simulink model "X8_trim"  (R2020a)
settings: Solver=ode45  StartTime=0.0  StopTime=20.0  RelTol=1e-4  EnableMultiTasking=on
values from neighbouring files (symbols this model uses):
  C_L_delta_eInterpolation = Create_interpolation(C_L_delta_e_data,'C_L_delta_e_data')    [coeff_ctrl.m]
  P = filter.P(i,i,k_0:k_1)    [filterTest.m]    (also in kalmanFilters.m = oldFilter.P(:,:,k))
  T_elevon2ailelev = [1 1 ... (first row only)    [init.m]
  x0 = X_trim    [X8Trim.m]    (also in init.m = [eta_0', ny_0' zeros(1,6)]'; runX8.m = [      0                 0                    -h_ini        ; trimX8.m = [      37.5                 0                    -h_ini     )
libraries: aerolibactuator x3
settings Model: Creator=krisgry  LastModifiedBy=olema
settings DataIOCC: LimitDataPoints=on  SaveFormat=Array  ReturnWorkspaceOutputs=off
settings OptimizationCC: LifeSpan=inf
settings DebuggingCC: SolverPrmCheckMsg=warning  SFUnexpectedBacktrackingDiag=warning  SFNoUnconditionalDefaultTransitionDiag=warning  SFExecutionAtInitializationDiag=none  UnderSpecifiedDimensionMsg=warning  ArithmeticOperatorsInVariantConditions=warning
settings HardwareCC: ProdBitPerPointer=32  ProdBitPerSizeT=32  ProdBitPerPtrDiffT=32  ProdLargestAtomicFloat=None  ProdIntDivRoundTo=Undefined  ProdEndianess=Unspecified  ProdWordSize=32  ProdHWDeviceType=32-bit Generic
settings ModelReferenceCC: PropagateSignalLabelsOutOfModel=off
settings SFSimCC: SimUseLocalCustomCode=off  CustomCodeUndefinedFunction=UseInterfaceOnly
settings RTWCC: RTWUseLocalCustomCode=off
settings CodeAppCC: StateflowObjectComments=on
settings GRTTargetCC: TargetLangStandard=C89/C90 (ANSI)
settings ConfigComp: CovMetricSettings=dw  CovHtmlReporting=on  CovSaveCumulativeToWorkspaceVar=on  CovSaveSingleToWorkspaceVar=on  CovExternalEMLEnable=off  CovSFcnEnable=off

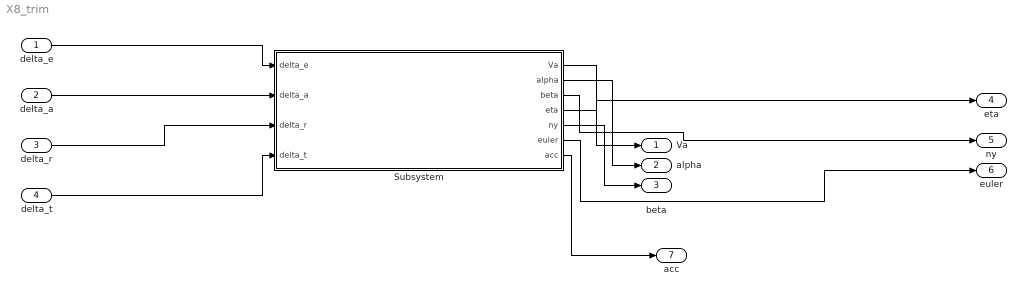
== system X8_trim ==
  delta_e : Inport
  delta_a : Inport  Port=2
  delta_r : Inport  Port=3
  delta_t : Inport  Port=4
  Subsystem : Subsystem
  Va : Outport  VectorParamsAs1DForOutWhenUnconnected=off
  alpha : Outport  Port=2  VectorParamsAs1DForOutWhenUnconnected=off
  beta : Outport  Port=3  VectorParamsAs1DForOutWhenUnconnected=off
  eta : Outport  Port=4  VectorParamsAs1DForOutWhenUnconnected=off
  ny : Outport  Port=5  VectorParamsAs1DForOutWhenUnconnected=off
  euler : Outport  Port=6  VectorParamsAs1DForOutWhenUnconnected=off
  acc : Outport  Port=7  VectorParamsAs1DForOutWhenUnconnected=off
  wires:
  delta_e/1 -> Subsystem/1(delta_e)
  delta_a/1 -> Subsystem/2(delta_a)
  delta_r/1 -> Subsystem/3(delta_r)
  delta_t/1 -> Subsystem/4(delta_t)
  Subsystem/1(Va) -> Va/1
  Subsystem/2(alpha) -> alpha/1
  Subsystem/3(beta) -> beta/1
  Subsystem/4(eta) -> eta/1
  Subsystem/5(ny) -> ny/1
  Subsystem/6(euler) -> euler/1
  Subsystem/7(acc) -> acc/1

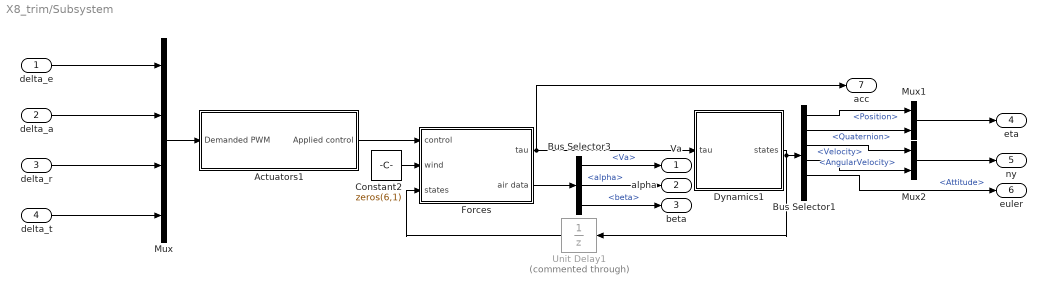
== system X8_trim/Subsystem ==
  delta_e : Inport
  delta_a : Inport  Port=2
  delta_r : Inport  Port=3
  delta_t : Inport  Port=4
  Actuators1 : Subsystem
  Bus Selector1 : BusSelector  OutputSignals=Position,Quaternion,Velocity,AngularVelocity,Attitude,Acceleration
  Bus Selector3 : BusSelector  OutputSignals=Va,alpha,beta
  Constant2 : Constant  Value=zeros(6,1)
  Dynamics1 : Subsystem
  Forces : Subsystem
  Mux : Mux
  Mux1 : Mux  Inputs=2
  Mux2 : Mux  Inputs=2
  Unit Delay1 : UnitDelay  Commented=through  SampleTime=-1  HasFrameUpgradeWarning=on
  Va : Outport  VectorParamsAs1DForOutWhenUnconnected=off
  alpha : Outport  Port=2  VectorParamsAs1DForOutWhenUnconnected=off
  beta : Outport  Port=3  VectorParamsAs1DForOutWhenUnconnected=off
  eta : Outport  Port=4  VectorParamsAs1DForOutWhenUnconnected=off
  ny : Outport  Port=5  VectorParamsAs1DForOutWhenUnconnected=off
  euler : Outport  Port=6  VectorParamsAs1DForOutWhenUnconnected=off
  acc : Outport  Port=7  VectorParamsAs1DForOutWhenUnconnected=off
  wires:
  Bus Selector3/2 -> alpha/1  "<alpha>"
  delta_a/1 -> Mux/2
  Bus Selector1/4 -> Mux2/2  "<AngularVelocity>"
  Constant2/1 -> Forces/2(wind)
  Bus Selector1/1 -> Mux1/1  "<Position>"
  delta_t/1 -> Mux/4
  Bus Selector3/3 -> beta/1  "<beta>"
  Forces/2(air data) -> Bus Selector3/1
  Mux2/1 -> ny/1
  Mux/1 -> Actuators1/1(Demanded PWM)
  Mux1/1 -> eta/1
  delta_r/1 -> Mux/3
  Dynamics1/1(states) -> Unit Delay1/1, Bus Selector1/1
  Bus Selector1/2 -> Mux1/2  "<Quaternion>"
  Actuators1/1(Applied control) -> Forces/1(control)
  Bus Selector1/5 -> euler/1  "<Attitude>"
  Bus Selector3/1 -> Va/1  "<Va>"
  Bus Selector1/3 -> Mux2/1  "<Velocity>"
  delta_e/1 -> Mux/1
  Unit Delay1/1 -> Forces/3(states)
  Forces/1(tau) -> acc/1, Dynamics1/1(tau)

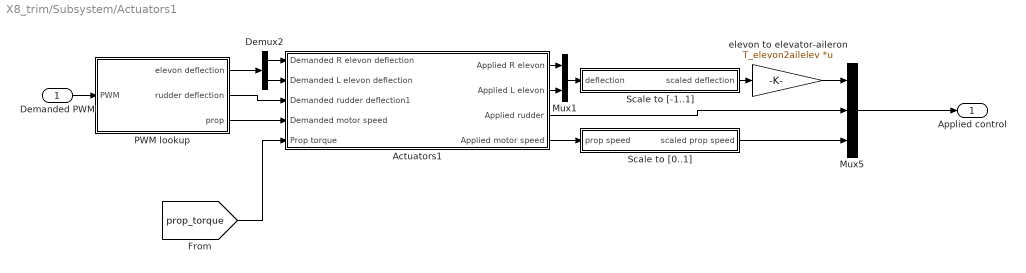
== system X8_trim/Subsystem/Actuators1 ==
  Demanded PWM : Inport
  Actuators1 : Subsystem
  Demux2 : Demux  Outputs=2
  Mux1 : Mux  Inputs=2
  Mux5 : Mux  Inputs=3
  PWM lookup : Subsystem
  Scale to [-1..1] : Subsystem
  Scale to [0..1] : Subsystem
  elevon to elevator-aileron : Gain  Gain=T_elevon2ailelev  Multiplication=Matrix(K*u) (u vector)
  Applied control : Outport  VectorParamsAs1DForOutWhenUnconnected=off
  wires:
  Demanded PWM/1 -> PWM lookup/1(PWM)
  PWM lookup/3("prop ") -> Actuators1/4(Demanded motor speed)
  Mux5/1 -> Applied control/1
  [prop_torque] -> Actuators1/5(Prop torque)
  Actuators1/4(Applied motor speed) -> Scale to [0..1]/1(prop speed)
  Scale to [-1..1]/1(scaled deflection) -> elevon to elevator-aileron/1
  elevon to elevator-aileron/1 -> Mux5/1
  PWM lookup/2(rudder deflection) -> Actuators1/3(Demanded rudder deflection1)
  Actuators1/3(Applied rudder) -> Mux5/2
  Scale to [0..1]/1(scaled prop speed) -> Mux5/3
  PWM lookup/1(elevon deflection) -> Demux2/1
  Demux2/1 -> Actuators1/1(Demanded R elevon deflection)
  Demux2/2 -> Actuators1/2("Demanded L elevon deflection ")
  Actuators1/1(Applied R elevon) -> Mux1/1
  Actuators1/2(Applied L elevon) -> Mux1/2
  Mux1/1 -> Scale to [-1..1]/1(deflection)

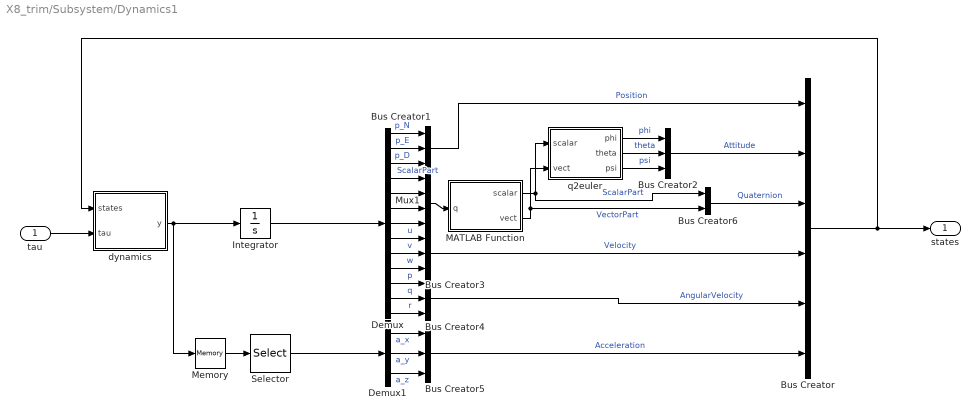
== system X8_trim/Subsystem/Dynamics1 ==
  tau : Inport
  Bus Creator : BusCreator  Inputs=6  OutDataTypeStr=Bus: States
  Bus Creator1 : BusCreator  Inputs=3  OutDataTypeStr=Bus: Position
  Bus Creator2 : BusCreator  Inputs=3  OutDataTypeStr=Bus: Attitude
  Bus Creator3 : BusCreator  Inputs=3  OutDataTypeStr=Bus: Velocity
  Bus Creator4 : BusCreator  Inputs=3  OutDataTypeStr=Bus: AngularVelocity
  Bus Creator5 : BusCreator  Inputs=3  OutDataTypeStr=Bus: Acceleration
  Bus Creator6 : BusCreator  Inputs=2  OutDataTypeStr=Bus: Quaternion
  Demux : Demux  Outputs=13
  Demux1 : Demux  Outputs=3
  Integrator : Integrator  InitialCondition=x0(1:13)
  MATLAB Function : MATLAB Function  TreatAsAtomicUnit=on
  Memory : Memory
  Mux1 : Mux
  Selector : Selector  InputPortWidth=13  IndexOptions=Index vector (dialog)  Indices=8:10  OutputSizes=1
  dynamics : MATLAB Function  TreatAsAtomicUnit=on
  q2euler : MATLAB Function  TreatAsAtomicUnit=on
  states : Outport  VectorParamsAs1DForOutWhenUnconnected=off
  wires:
  dynamics/1(y) -> Memory/1, Integrator/1
  tau/1 -> dynamics/2(tau)
  Bus Creator/1 -> states/1, dynamics/1(states)
  Demux/2 -> Bus Creator1/2  "p_E"
  Demux/3 -> Bus Creator1/3  "p_D"
  Demux/1 -> Bus Creator1/1  "p_N"
  q2euler/2(theta) -> Bus Creator2/2  "theta"
  q2euler/3(psi) -> Bus Creator2/3  "psi"
  q2euler/1(phi) -> Bus Creator2/1  "phi"
  Demux/10 -> Bus Creator3/3  "w"
  Demux/8 -> Bus Creator3/1  "u"
  Demux/9 -> Bus Creator3/2  "v"
  Demux/11 -> Bus Creator4/1  "p"
  Demux/13 -> Bus Creator4/3  "r"
  Demux/12 -> Bus Creator4/2  "q"
  Bus Creator3/1 -> Bus Creator/4  "Velocity"
  Bus Creator1/1 -> Bus Creator/1  "Position"
  Bus Creator4/1 -> Bus Creator/5  "AngularVelocity"
  Bus Creator5/1 -> Bus Creator/6  "Acceleration"
  Selector/1 -> Demux1/1
  Demux1/1 -> Bus Creator5/1  "a_x"
  Demux1/2 -> Bus Creator5/2  "a_y"
  Demux1/3 -> Bus Creator5/3  "a_z"
  Demux/6 -> Mux1/3
  Demux/7 -> Mux1/4
  Demux/5 -> Mux1/2
  Integrator/1 -> Demux/1
  MATLAB Function/1(scalar) -> Bus Creator6/1, q2euler/1(scalar)  "ScalarPart"
  MATLAB Function/2(vect) -> Bus Creator6/2, q2euler/2(vect)  "VectorPart"
  Bus Creator6/1 -> Bus Creator/3  "Quaternion"
  Demux/4 -> Mux1/1  "ScalarPart"
  Bus Creator2/1 -> Bus Creator/2  "Attitude"
  Mux1/1 -> MATLAB Function/1(q)
  Memory/1 -> Selector/1

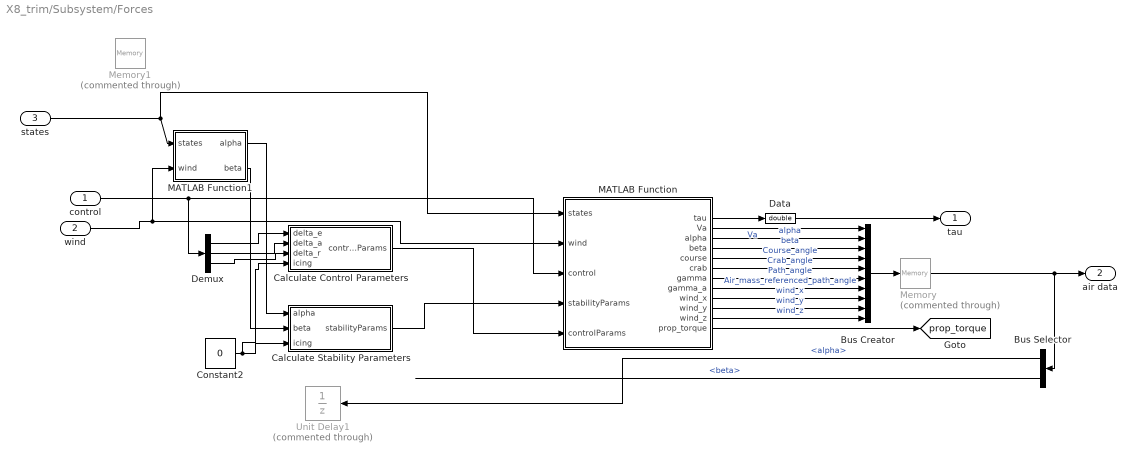
== system X8_trim/Subsystem/Forces ==
  control : Inport
  wind : Inport  Port=2
  states : Inport  Port=3
  Bus Creator : BusCreator  Inputs=10  OutDataTypeStr=Bus: AirData
  Bus Selector : BusSelector  OutputSignals=alpha,beta
  Calculate Control Parameters : Subsystem
  Calculate Stability Parameters : Subsystem
  Constant2 : Constant  Value=0
  Data : DataTypeConversion  OutDataTypeStr=double
  Demux : Demux  Outputs=3
  MATLAB Function : MATLAB Function  TreatAsAtomicUnit=on
  MATLAB Function1 : MATLAB Function  TreatAsAtomicUnit=on
  Memory : Memory  Commented=through  InitialCondition=1e-15
  Memory1 : Memory  Commented=through  InitialCondition=1e-15
  Unit Delay1 : UnitDelay  Commented=through  SampleTime=-1  HasFrameUpgradeWarning=on
  tau : Outport  VectorParamsAs1DForOutWhenUnconnected=off
  air data : Outport  Port=2  VectorParamsAs1DForOutWhenUnconnected=off
  tag scope: prop_torque=global
  wires:
  control/1 -> Demux/1, MATLAB Function/3(control)
  wind/1 -> MATLAB Function1/2(wind), MATLAB Function/2(wind)
  MATLAB Function/1(tau) -> Data/1
  MATLAB Function/12(prop_torque) -> [prop_torque]
  Memory/1 -> Bus Selector/1, air data/1
  Bus Creator/1 -> Memory/1
  MATLAB Function/11(wind_z) -> Bus Creator/10  "wind_z"
  MATLAB Function/10(wind_y) -> Bus Creator/9  "wind_y"
  MATLAB Function/9(wind_x) -> Bus Creator/8  "wind_x"
  MATLAB Function/8(gamma_a) -> Bus Creator/7  "Air_mass_referenced_path_angle"
  MATLAB Function/7(gamma) -> Bus Creator/6  "Path_angle"
  MATLAB Function/6(crab) -> Bus Creator/5  "Crab_angle"
  MATLAB Function/5(course) -> Bus Creator/4  "Course_angle"
  MATLAB Function/4(beta) -> Bus Creator/3  "beta"
  MATLAB Function/3(alpha) -> Bus Creator/2  "alpha"
  MATLAB Function/2(Va) -> Bus Creator/1  "Va"
  Data/1 -> tau/1
  Constant2/1 -> Calculate Control Parameters/4(icing), Calculate Stability Parameters/3(icing)
  Calculate Stability Parameters/1(stabilityParams) -> MATLAB Function/4(stabilityParams)
  Bus Selector/1 -> Unit Delay1/1  "<alpha>"
  Bus Selector/2 -> ?  "<beta>"
  Demux/1 -> Calculate Control Parameters/1("delta_e ")
  Demux/2 -> Calculate Control Parameters/2(delta_a)
  Demux/3 -> Calculate Control Parameters/3("delta_r ")
  Calculate Control Parameters/1(controlParams) -> MATLAB Function/5(controlParams)
  MATLAB Function1/1(alpha) -> Calculate Stability Parameters/1("alpha ")
  MATLAB Function1/2(beta) -> Calculate Stability Parameters/2(beta)
  states/1 -> MATLAB Function/1(states), MATLAB Function1/1(states)

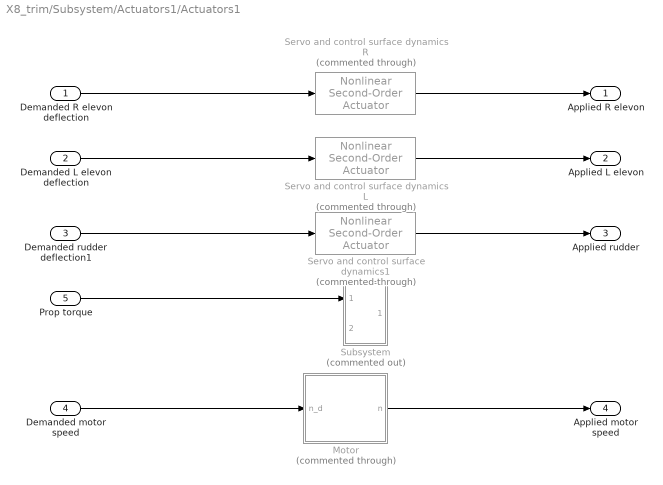
== system X8_trim/Subsystem/Actuators1/Actuators1 ==
  Demanded R elevon deflection : Inport
  "Demanded L elevon deflection " : Inport  Port=2
  Demanded rudder deflection1 : Inport  Port=3
  Demanded motor speed : Inport  Port=4
  Prop torque : Inport  Port=5
  Motor : Subsystem  Commented=through  mask{T=0.2, X0=x0(18)}
      mask prompts: T "Time constant"; X0 "Initial condition"
      mask DialogControl DescGroupVar Prompt: Motor model
      mask DialogControl DescTextVar Prompt: Simple first order motor model
  Servo and control surface dynamics L : aerolibactuator/Nonlinear Second-Order Actuator  Commented=through  wn_fin=P.servo.omega0  z_fin=P.servo.zeta  fin_max=P.servo.max_rad  fin_min=P.servo.min_rad  fin_maxrate=P.servo.rate_lim  fin_act_0=x0(16)  fin_act_vel=x0(17)
      settings: SourceProductBaseCode=AE
  Servo and control surface dynamics R : aerolibactuator/Nonlinear Second-Order Actuator  Commented=through  wn_fin=P.servo.omega0  z_fin=P.servo.zeta  fin_max=P.servo.max_rad  fin_min=P.servo.min_rad  fin_maxrate=P.servo.rate_lim  fin_act_0=x0(14)  fin_act_vel=x0(15)
      settings: SourceProductBaseCode=AE
  Servo and control surface dynamics1 : aerolibactuator/Nonlinear Second-Order Actuator  Commented=through  wn_fin=P.servo.omega0  z_fin=P.servo.zeta  fin_max=P.servo.max_rad  fin_min=P.servo.min_rad  fin_maxrate=P.servo.rate_lim  fin_act_0=P.servo.pos0  fin_act_vel=P.servo.rate0
      settings: SourceProductBaseCode=AE
  Subsystem : Subsystem  Commented=on
  Applied R elevon : Outport  VectorParamsAs1DForOutWhenUnconnected=off
  Applied L elevon : Outport  Port=2  VectorParamsAs1DForOutWhenUnconnected=off
  Applied rudder : Outport  Port=3  VectorParamsAs1DForOutWhenUnconnected=off
  Applied motor speed : Outport  Port=4  VectorParamsAs1DForOutWhenUnconnected=off
  wires:
  Demanded R elevon deflection/1 -> Servo and control surface dynamics R/1
  Servo and control surface dynamics R/1 -> Applied R elevon/1
  Prop torque/1 -> Subsystem/1(In1)
  Demanded motor speed/1 -> Motor/1(n_d)
  Motor/1(n) -> Applied motor speed/1
  Demanded rudder deflection1/1 -> Servo and control surface dynamics1/1
  Servo and control surface dynamics1/1 -> Applied rudder/1
  "Demanded L elevon deflection "/1 -> Servo and control surface dynamics L/1
  Servo and control surface dynamics L/1 -> Applied L elevon/1

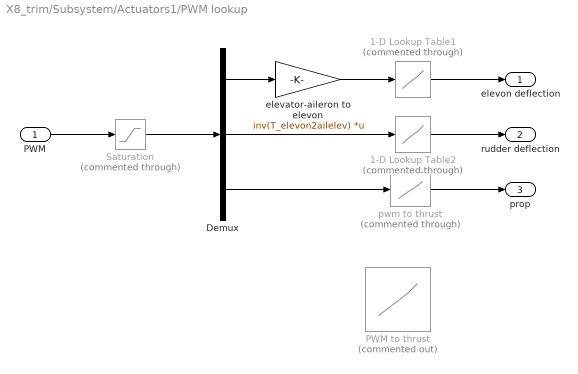
== system X8_trim/Subsystem/Actuators1/PWM lookup ==
  PWM : Inport
  1-D Lookup Table1 : Lookup_n-D  Commented=through  NumberOfTableDimensions=1  BreakpointsForDimension1=|  Table=|  InternalRulePriority=Speed  RndMeth=Simplest  InputSameDT=on
      BreakpointsForDimension1=|
      | [-20
      | -15
      | -10
      | 15
      | 20
      | 21.6]
      Table=|
      | [1260
      | 1400
      | 1480
      | 1770
      | 1880
      | 1920]
  1-D Lookup Table2 : Lookup_n-D  Commented=through  NumberOfTableDimensions=1  BreakpointsForDimension1=|  Table=|  InternalRulePriority=Speed  RndMeth=Simplest  InputSameDT=on
      BreakpointsForDimension1=|
      | [-20
      | -15
      | -10
      | 15
      | 20
      | 21.6]
      Table=|
      | [1260
      | 1400
      | 1480
      | 1770
      | 1880
      | 1920]
  Demux : Demux  Outputs=[2,1,1]
  PWM to thrust : Lookup_n-D  Commented=on  NumberOfTableDimensions=1  BreakpointsForDimension1=[1000, 2000]  Table=[0 1.700*9.81]  InternalRulePriority=Speed  RndMeth=Simplest  InputSameDT=on
  Saturation : Saturate  Commented=through  UpperLimit=P.pwmMax  LowerLimit=P.pwmMin
  elevator-aileron to elevon : Gain  Gain=inv(T_elevon2ailelev)  Multiplication=Matrix(K*u) (u vector)
  pwm to thrust : Lookup_n-D  Commented=through  NumberOfTableDimensions=1  BreakpointsForDimension1=[1000 2000]  Table=[0 1]  InternalRulePriority=Speed  RndMeth=Simplest  InputSameDT=on
  elevon deflection : Outport  VectorParamsAs1DForOutWhenUnconnected=off
  rudder deflection : Outport  Port=2  VectorParamsAs1DForOutWhenUnconnected=off
  "prop " : Outport  Port=3  VectorParamsAs1DForOutWhenUnconnected=off
  wires:
  pwm to thrust/1 -> "prop "/1
  PWM/1 -> Saturation/1
  Saturation/1 -> Demux/1
  Demux/1 -> elevator-aileron to elevon/1
  1-D Lookup Table1/1 -> elevon deflection/1
  elevator-aileron to elevon/1 -> 1-D Lookup Table1/1
  Demux/3 -> pwm to thrust/1
  Demux/2 -> 1-D Lookup Table2/1
  1-D Lookup Table2/1 -> rudder deflection/1

== system X8_trim/Subsystem/Actuators1/Scale to [-1..1] ==
  deflection : Inport
  Gain : Gain  Gain=P.rad2unit
  Saturation : Saturate  UpperLimit=1  LowerLimit=-1
  scaled deflection : Outport  VectorParamsAs1DForOutWhenUnconnected=off
  wires:
  deflection/1 -> Gain/1
  Gain/1 -> Saturation/1
  Saturation/1 -> scaled deflection/1

== system X8_trim/Subsystem/Actuators1/Scale to [0..1] ==
  prop speed : Inport
  Gain : Gain  Commented=through  Gain=1/P.motor.omega_max
  Saturation : Saturate  UpperLimit=1  LowerLimit=0
  scaled prop speed : Outport  VectorParamsAs1DForOutWhenUnconnected=off
  wires:
  prop speed/1 -> Gain/1
  Gain/1 -> Saturation/1
  Saturation/1 -> scaled prop speed/1

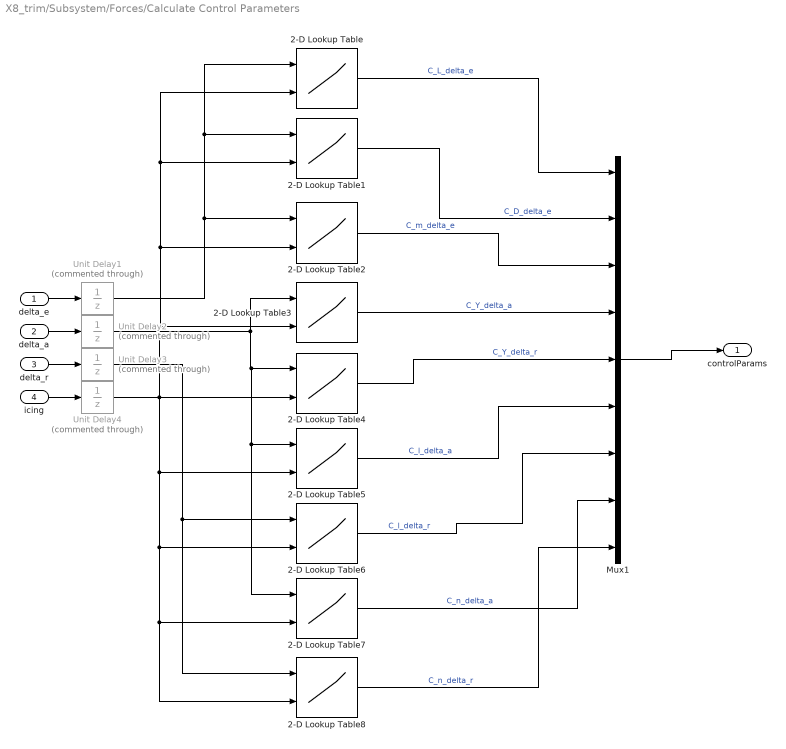
== system X8_trim/Subsystem/Forces/Calculate Control Parameters ==
  "delta_e " : Inport
  delta_a : Inport  Port=2
  "delta_r " : Inport  Port=3
  icing : Inport  Port=4
  2-D Lookup Table : Lookup_n-D  DataSpecification=Lookup table object  LookupTableObject=C_L_delta_eInterpolation  BreakpointsForDimension1=C_L_delta_eInterpolation.Points(:,1)  BreakpointsForDimension2=C_L_delta_eInterpolation.Points(:,2)  BreakpointsForDimension1FirstPoint=4  BreakpointsForDimension2FirstPoint=2  IndexSearchMethod=Linear search  Table=C_L_delta_eInterpolation.Values  ExtrapMethod=Clip  InternalRulePriority=Speed  RndMeth=Simplest  InputSameDT=on
  2-D Lookup Table1 : Lookup_n-D  DataSpecification=Lookup table object  LookupTableObject=C_D_delta_eInterpolation  BreakpointsForDimension1=C_L_delta_eInterpolation.Points(:,1)  BreakpointsForDimension2=C_L_delta_eInterpolation.Points(:,2)  BreakpointsForDimension1FirstPoint=4  BreakpointsForDimension2FirstPoint=2  IndexSearchMethod=Linear search  Table=C_L_delta_eInterpolation.Values  ExtrapMethod=Clip  InternalRulePriority=Speed  RndMeth=Simplest  InputSameDT=on
  2-D Lookup Table2 : Lookup_n-D  DataSpecification=Lookup table object  LookupTableObject=C_m_delta_eInterpolation  BreakpointsForDimension1=C_L_delta_eInterpolation.Points(:,1)  BreakpointsForDimension2=C_L_delta_eInterpolation.Points(:,2)  BreakpointsForDimension1FirstPoint=4  BreakpointsForDimension2FirstPoint=2  IndexSearchMethod=Linear search  Table=C_L_delta_eInterpolation.Values  ExtrapMethod=Clip  InternalRulePriority=Speed  RndMeth=Simplest  InputSameDT=on
  2-D Lookup Table3 : Lookup_n-D  DataSpecification=Lookup table object  LookupTableObject=C_Y_delta_aInterpolation  BreakpointsForDimension1=C_L_delta_eInterpolation.Points(:,1)  BreakpointsForDimension2=C_L_delta_eInterpolation.Points(:,2)  BreakpointsForDimension1FirstPoint=4  BreakpointsForDimension2FirstPoint=2  IndexSearchMethod=Linear search  Table=C_L_delta_eInterpolation.Values  ExtrapMethod=Clip  InternalRulePriority=Speed  RndMeth=Simplest  InputSameDT=on
  2-D Lookup Table4 : Lookup_n-D  DataSpecification=Lookup table object  LookupTableObject=C_Y_delta_rInterpolation  BreakpointsForDimension1=C_L_delta_eInterpolation.Points(:,1)  BreakpointsForDimension2=C_L_delta_eInterpolation.Points(:,2)  BreakpointsForDimension1FirstPoint=4  BreakpointsForDimension2FirstPoint=2  IndexSearchMethod=Linear search  Table=C_L_delta_eInterpolation.Values  ExtrapMethod=Clip  InternalRulePriority=Speed  RndMeth=Simplest  InputSameDT=on
  2-D Lookup Table5 : Lookup_n-D  DataSpecification=Lookup table object  LookupTableObject=C_l_delta_aInterpolation  BreakpointsForDimension1=C_L_delta_eInterpolation.Points(:,1)  BreakpointsForDimension2=C_L_delta_eInterpolation.Points(:,2)  BreakpointsForDimension1FirstPoint=4  BreakpointsForDimension2FirstPoint=2  IndexSearchMethod=Linear search  Table=C_L_delta_eInterpolation.Values  ExtrapMethod=Clip  InternalRulePriority=Speed  RndMeth=Simplest  InputSameDT=on
  2-D Lookup Table6 : Lookup_n-D  DataSpecification=Lookup table object  LookupTableObject=C_l_delta_rInterpolation  BreakpointsForDimension1=C_L_delta_eInterpolation.Points(:,1)  BreakpointsForDimension2=C_L_delta_eInterpolation.Points(:,2)  BreakpointsForDimension1FirstPoint=4  BreakpointsForDimension2FirstPoint=2  IndexSearchMethod=Linear search  Table=C_L_delta_eInterpolation.Values  ExtrapMethod=Clip  InternalRulePriority=Speed  RndMeth=Simplest  InputSameDT=on
  2-D Lookup Table7 : Lookup_n-D  DataSpecification=Lookup table object  LookupTableObject=C_n_delta_aInterpolation  BreakpointsForDimension1=C_L_delta_eInterpolation.Points(:,1)  BreakpointsForDimension2=C_L_delta_eInterpolation.Points(:,2)  BreakpointsForDimension1FirstPoint=4  BreakpointsForDimension2FirstPoint=2  IndexSearchMethod=Linear search  Table=C_L_delta_eInterpolation.Values  ExtrapMethod=Clip  InternalRulePriority=Speed  RndMeth=Simplest  InputSameDT=on
  2-D Lookup Table8 : Lookup_n-D  DataSpecification=Lookup table object  LookupTableObject=C_n_delta_rInterpolation  BreakpointsForDimension1=C_L_delta_eInterpolation.Points(:,1)  BreakpointsForDimension2=C_L_delta_eInterpolation.Points(:,2)  BreakpointsForDimension1FirstPoint=4  BreakpointsForDimension2FirstPoint=2  IndexSearchMethod=Linear search  Table=C_L_delta_eInterpolation.Values  ExtrapMethod=Clip  InternalRulePriority=Speed  RndMeth=Simplest  InputSameDT=on
  Mux1 : Mux  Inputs=9
  Unit Delay{1..4} (4 alike) : UnitDelay  Commented=through  SampleTime=-1  HasFrameUpgradeWarning=on
  controlParams : Outport  VectorParamsAs1DForOutWhenUnconnected=off
  wires:
  Mux1/1 -> controlParams/1
  "delta_e "/1 -> Unit Delay1/1
  delta_a/1 -> Unit Delay2/1
  "delta_r "/1 -> Unit Delay3/1
  icing/1 -> Unit Delay4/1
  2-D Lookup Table/1 -> Mux1/1  "C_L_delta_e"
  2-D Lookup Table8/1 -> Mux1/9  "C_n_delta_r"
  2-D Lookup Table1/1 -> Mux1/2  "C_D_delta_e"
  2-D Lookup Table2/1 -> Mux1/3  "C_m_delta_e"
  2-D Lookup Table3/1 -> Mux1/4  "C_Y_delta_a"
  2-D Lookup Table4/1 -> Mux1/5  "C_Y_delta_r"
  2-D Lookup Table5/1 -> Mux1/6  "C_l_delta_a"
  2-D Lookup Table6/1 -> Mux1/7  "C_l_delta_r"
  2-D Lookup Table7/1 -> Mux1/8  "C_n_delta_a"
  Unit Delay1/1 -> 2-D Lookup Table2/1, 2-D Lookup Table1/1, 2-D Lookup Table/1
  Unit Delay2/1 -> 2-D Lookup Table3/1, 2-D Lookup Table7/1, 2-D Lookup Table5/1, 2-D Lookup Table4/1
  Unit Delay3/1 -> 2-D Lookup Table8/1, 2-D Lookup Table6/1
  Unit Delay4/1 -> 2-D Lookup Table/2, 2-D Lookup Table1/2, 2-D Lookup Table2/2, 2-D Lookup Table3/2, 2-D Lookup Table5/2, 2-D Lookup Table6/2, 2-D Lookup Table7/2, 2-D Lookup Table8/2, 2-D Lookup Table4/2

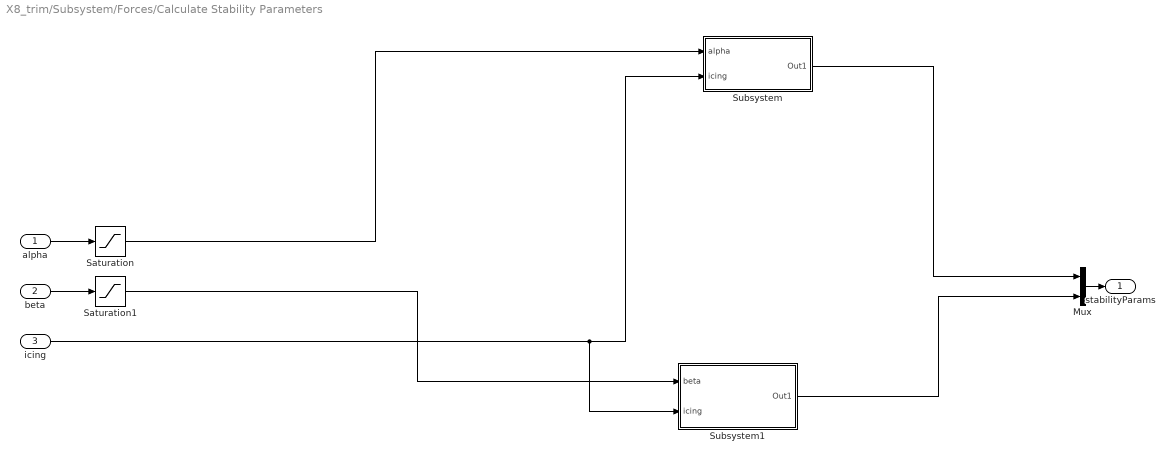
== system X8_trim/Subsystem/Forces/Calculate Stability Parameters ==
  "alpha " : Inport
  beta : Inport  Port=2
  icing : Inport  Port=3
  Mux : Mux  Inputs=2
  Saturation : Saturate  UpperLimit=deg2rad(15)  LowerLimit=deg2rad(-10)
  Saturation1 : Saturate  UpperLimit=deg2rad(15)  LowerLimit=deg2rad(-15)
  Subsystem : Subsystem
  Subsystem1 : Subsystem
  stabilityParams : Outport  VectorParamsAs1DForOutWhenUnconnected=off
  wires:
  "alpha "/1 -> Saturation/1
  beta/1 -> Saturation1/1
  Saturation/1 -> Subsystem/1(alpha)
  icing/1 -> Subsystem1/2(icing), Subsystem/2(icing)
  Subsystem1/1(Out1) -> Mux/2
  Subsystem/1(Out1) -> Mux/1
  Saturation1/1 -> Subsystem1/1(beta)
  Mux/1 -> stabilityParams/1

== system X8_trim/Subsystem/Actuators1/Actuators1/Motor ==
  n_d : Inport
  1/T : Gain  Gain=1/T
  Integrator : Integrator  InitialCondition=X0  ContinuousStateAttributes='throttle'
  Sum : Sum  Inputs=|+-
  n : Outport  VectorParamsAs1DForOutWhenUnconnected=off
  wires:
  Integrator/1 -> n/1, Sum/2
  n_d/1 -> Sum/1
  Sum/1 -> 1/T/1
  1/T/1 -> Integrator/1

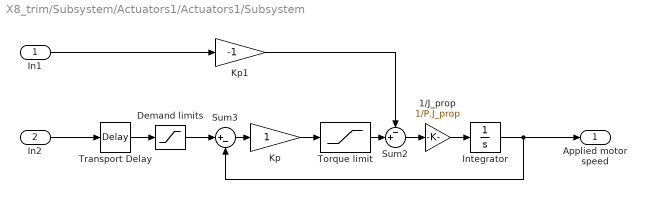
== system X8_trim/Subsystem/Actuators1/Actuators1/Subsystem ==
  In1 : Inport
  In2 : Inport  Port=2
  1/J_prop : Gain  Gain=1/P.J_prop  SaturateOnIntegerOverflow=on  OutDataTypeStr=Inherit: Same as input  ParamDataTypeStr=Inherit: Same as input
  Demand limits : Saturate  UpperLimit=1  LowerLimit=0
  Integrator : Integrator  InitialCondition=0.5
  Kp : Gain  SaturateOnIntegerOverflow=on  OutDataTypeStr=Inherit: Same as input  ParamDataTypeStr=Inherit: Same as input
  Kp1 : Gain  Gain=-1  SaturateOnIntegerOverflow=on  OutDataTypeStr=Inherit: Same as input  ParamDataTypeStr=Inherit: Same as input
  Sum2 : Sum  Inputs=-+|  InputSameDT=on  SaturateOnIntegerOverflow=on  OutDataTypeStr=Inherit: Same as first input
  Sum3 : Sum  Inputs=|+-  InputSameDT=on  SaturateOnIntegerOverflow=on  OutDataTypeStr=Inherit: Same as first input
  Torque limit : Saturate  UpperLimit=P.motor.torque_max  LowerLimit=0  ZeroCross=off
  Transport Delay : TransportDelay  DelayTime=0.001  PadeOrder=1
  Applied motor speed : Outport  VectorParamsAs1DForOutWhenUnconnected=off
  wires:
  Demand limits/1 -> Sum3/1
  Sum3/1 -> Kp/1
  Integrator/1 -> Applied motor speed/1, Sum3/2
  Torque limit/1 -> Sum2/2
  Sum2/1 -> 1/J_prop/1
  1/J_prop/1 -> Integrator/1
  Kp/1 -> Torque limit/1
  In1/1 -> Kp1/1
  In2/1 -> Transport Delay/1
  Transport Delay/1 -> Demand limits/1
  Kp1/1 -> Sum2/1

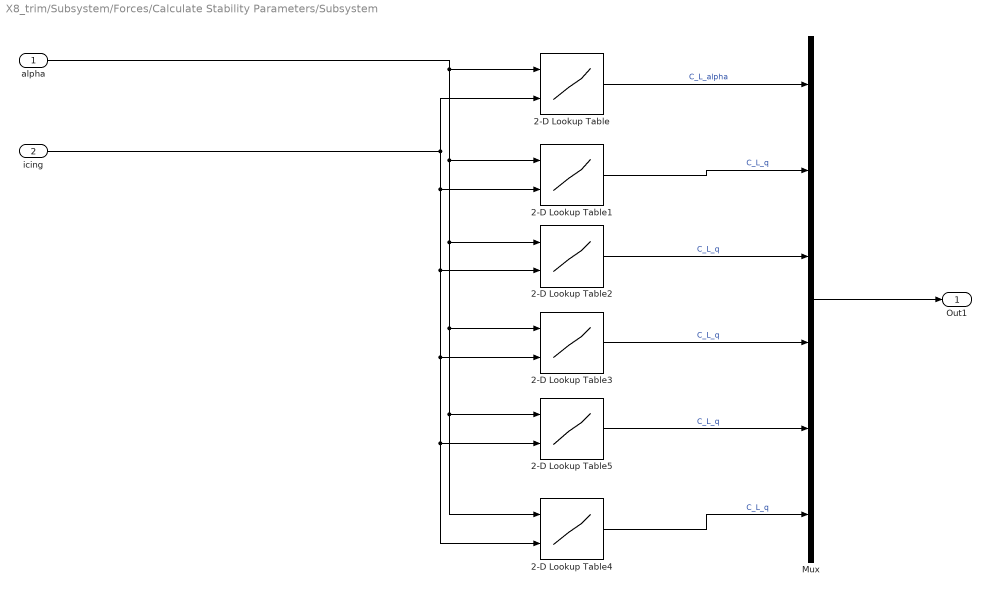
== system X8_trim/Subsystem/Forces/Calculate Stability Parameters/Subsystem ==
  alpha : Inport
  icing : Inport  Port=2
  2-D Lookup Table : Lookup_n-D  DataSpecification=Lookup table object  LookupTableObject=C_L_aInterpolation  BreakpointsForDimension1=C_L_delta_eInterpolation.Points(:,1)  BreakpointsForDimension2=C_L_delta_eInterpolation.Points(:,2)  BreakpointsForDimension1FirstPoint=4  BreakpointsForDimension2FirstPoint=2  IndexSearchMethod=Linear search  Table=C_L_delta_eInterpolation.Values  InterpMethod=Linear Lagrange  InternalRulePriority=Speed  RndMeth=Simplest  InputSameDT=on
  2-D Lookup Table1 : Lookup_n-D  DataSpecification=Lookup table object  LookupTableObject=C_L_qInterpolation  BreakpointsForDimension1=C_L_delta_eInterpolation.Points(:,1)  BreakpointsForDimension2=C_L_delta_eInterpolation.Points(:,2)  BreakpointsForDimension1FirstPoint=4  BreakpointsForDimension2FirstPoint=2  IndexSearchMethod=Linear search  Table=C_L_delta_eInterpolation.Values  InternalRulePriority=Speed  RndMeth=Simplest  InputSameDT=on
  2-D Lookup Table2 : Lookup_n-D  DataSpecification=Lookup table object  LookupTableObject=C_D_aInterpolation  BreakpointsForDimension1=C_L_delta_eInterpolation.Points(:,1)  BreakpointsForDimension2=C_L_delta_eInterpolation.Points(:,2)  BreakpointsForDimension1FirstPoint=4  BreakpointsForDimension2FirstPoint=2  IndexSearchMethod=Linear search  Table=C_L_delta_eInterpolation.Values  InternalRulePriority=Speed  RndMeth=Simplest  InputSameDT=on
  2-D Lookup Table3 : Lookup_n-D  DataSpecification=Lookup table object  LookupTableObject=C_D_qInterpolation  BreakpointsForDimension1=C_L_delta_eInterpolation.Points(:,1)  BreakpointsForDimension2=C_L_delta_eInterpolation.Points(:,2)  BreakpointsForDimension1FirstPoint=4  BreakpointsForDimension2FirstPoint=2  IndexSearchMethod=Linear search  Table=C_L_delta_eInterpolation.Values  InternalRulePriority=Speed  RndMeth=Simplest  InputSameDT=on
  2-D Lookup Table4 : Lookup_n-D  DataSpecification=Lookup table object  LookupTableObject=C_m_qInterpolation  BreakpointsForDimension1=C_L_delta_eInterpolation.Points(:,1)  BreakpointsForDimension2=C_L_delta_eInterpolation.Points(:,2)  BreakpointsForDimension1FirstPoint=4  BreakpointsForDimension2FirstPoint=2  IndexSearchMethod=Linear search  Table=C_L_delta_eInterpolation.Values  InternalRulePriority=Speed  RndMeth=Simplest  InputSameDT=on
  2-D Lookup Table5 : Lookup_n-D  DataSpecification=Lookup table object  LookupTableObject=C_m_aInterpolation  BreakpointsForDimension1=C_L_delta_eInterpolation.Points(:,1)  BreakpointsForDimension2=C_L_delta_eInterpolation.Points(:,2)  BreakpointsForDimension1FirstPoint=4  BreakpointsForDimension2FirstPoint=2  IndexSearchMethod=Linear search  Table=C_L_delta_eInterpolation.Values  InternalRulePriority=Speed  RndMeth=Simplest  InputSameDT=on
  Mux : Mux  Inputs=6
  Out1 : Outport  VectorParamsAs1DForOutWhenUnconnected=off
  wires:
  Mux/1 -> Out1/1
  2-D Lookup Table/1 -> Mux/1  "C_L_alpha"
  alpha/1 -> 2-D Lookup Table4/1, 2-D Lookup Table5/1, 2-D Lookup Table3/1, 2-D Lookup Table2/1, 2-D Lookup Table1/1, 2-D Lookup Table/1
  icing/1 -> 2-D Lookup Table3/2, 2-D Lookup Table5/2, 2-D Lookup Table4/2, 2-D Lookup Table2/2, 2-D Lookup Table1/2, 2-D Lookup Table/2
  2-D Lookup Table1/1 -> Mux/2  "C_L_q"
  2-D Lookup Table2/1 -> Mux/3  "C_L_q"
  2-D Lookup Table3/1 -> Mux/4  "C_L_q"
  2-D Lookup Table5/1 -> Mux/5  "C_L_q"
  2-D Lookup Table4/1 -> Mux/6  "C_L_q"

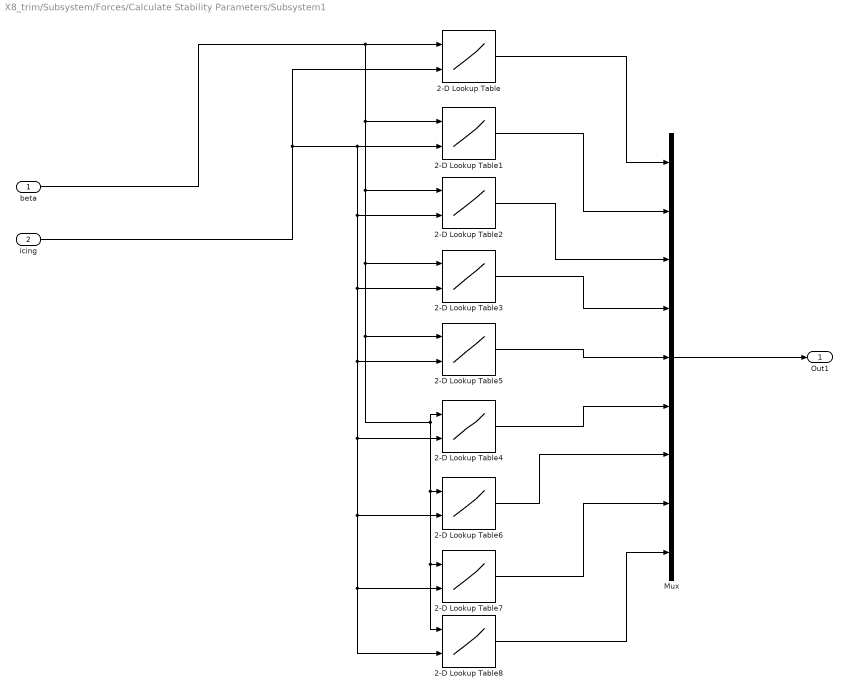
== system X8_trim/Subsystem/Forces/Calculate Stability Parameters/Subsystem1 ==
  beta : Inport
  icing : Inport  Port=2
  2-D Lookup Table : Lookup_n-D  DataSpecification=Lookup table object  LookupTableObject=C_Y_bInterpolation  BreakpointsForDimension1=C_L_delta_eInterpolation.Points(:,1)  BreakpointsForDimension2=C_L_delta_eInterpolation.Points(:,2)  BreakpointsForDimension1FirstPoint=4  BreakpointsForDimension2FirstPoint=2  IndexSearchMethod=Linear search  Table=C_L_delta_eInterpolation.Values  InternalRulePriority=Speed  RndMeth=Simplest  InputSameDT=on
  2-D Lookup Table1 : Lookup_n-D  DataSpecification=Lookup table object  LookupTableObject=C_Y_pInterpolation  BreakpointsForDimension1=C_L_delta_eInterpolation.Points(:,1)  BreakpointsForDimension2=C_L_delta_eInterpolation.Points(:,2)  BreakpointsForDimension1FirstPoint=4  BreakpointsForDimension2FirstPoint=2  IndexSearchMethod=Linear search  Table=C_L_delta_eInterpolation.Values  InternalRulePriority=Speed  RndMeth=Simplest  InputSameDT=on
  2-D Lookup Table2 : Lookup_n-D  DataSpecification=Lookup table object  LookupTableObject=C_Y_rInterpolation  BreakpointsForDimension1=C_L_delta_eInterpolation.Points(:,1)  BreakpointsForDimension2=C_L_delta_eInterpolation.Points(:,2)  BreakpointsForDimension1FirstPoint=4  BreakpointsForDimension2FirstPoint=2  IndexSearchMethod=Linear search  Table=C_L_delta_eInterpolation.Values  InternalRulePriority=Speed  RndMeth=Simplest  InputSameDT=on
  2-D Lookup Table3 : Lookup_n-D  DataSpecification=Lookup table object  LookupTableObject=C_l_bInterpolation  BreakpointsForDimension1=C_L_delta_eInterpolation.Points(:,1)  BreakpointsForDimension2=C_L_delta_eInterpolation.Points(:,2)  BreakpointsForDimension1FirstPoint=4  BreakpointsForDimension2FirstPoint=2  IndexSearchMethod=Linear search  Table=C_L_delta_eInterpolation.Values  InternalRulePriority=Speed  RndMeth=Simplest  InputSameDT=on
  2-D Lookup Table4 : Lookup_n-D  DataSpecification=Lookup table object  LookupTableObject=C_l_rInterpolation  BreakpointsForDimension1=C_L_delta_eInterpolation.Points(:,1)  BreakpointsForDimension2=C_L_delta_eInterpolation.Points(:,2)  BreakpointsForDimension1FirstPoint=4  BreakpointsForDimension2FirstPoint=2  IndexSearchMethod=Linear search  Table=C_L_delta_eInterpolation.Values  InternalRulePriority=Speed  RndMeth=Simplest  InputSameDT=on
  2-D Lookup Table5 : Lookup_n-D  DataSpecification=Lookup table object  LookupTableObject=C_l_pInterpolation  BreakpointsForDimension1=C_L_delta_eInterpolation.Points(:,1)  BreakpointsForDimension2=C_L_delta_eInterpolation.Points(:,2)  BreakpointsForDimension1FirstPoint=4  BreakpointsForDimension2FirstPoint=2  IndexSearchMethod=Linear search  Table=C_L_delta_eInterpolation.Values  InternalRulePriority=Speed  RndMeth=Simplest  InputSameDT=on
  2-D Lookup Table6 : Lookup_n-D  DataSpecification=Lookup table object  LookupTableObject=C_n_bInterpolation  BreakpointsForDimension1=C_L_delta_eInterpolation.Points(:,1)  BreakpointsForDimension2=C_L_delta_eInterpolation.Points(:,2)  BreakpointsForDimension1FirstPoint=4  BreakpointsForDimension2FirstPoint=2  IndexSearchMethod=Linear search  Table=C_L_delta_eInterpolation.Values  InternalRulePriority=Speed  RndMeth=Simplest  InputSameDT=on
  2-D Lookup Table7 : Lookup_n-D  DataSpecification=Lookup table object  LookupTableObject=C_n_pInterpolation  BreakpointsForDimension1=C_L_delta_eInterpolation.Points(:,1)  BreakpointsForDimension2=C_L_delta_eInterpolation.Points(:,2)  BreakpointsForDimension1FirstPoint=4  BreakpointsForDimension2FirstPoint=2  IndexSearchMethod=Linear search  Table=C_L_delta_eInterpolation.Values  InternalRulePriority=Speed  RndMeth=Simplest  InputSameDT=on
  2-D Lookup Table8 : Lookup_n-D  DataSpecification=Lookup table object  LookupTableObject=C_n_rInterpolation  BreakpointsForDimension1=C_L_delta_eInterpolation.Points(:,1)  BreakpointsForDimension2=C_L_delta_eInterpolation.Points(:,2)  BreakpointsForDimension1FirstPoint=4  BreakpointsForDimension2FirstPoint=2  IndexSearchMethod=Linear search  Table=C_L_delta_eInterpolation.Values  InternalRulePriority=Speed  RndMeth=Simplest  InputSameDT=on
  Mux : Mux  Inputs=9
  Out1 : Outport  VectorParamsAs1DForOutWhenUnconnected=off
  wires:
  Mux/1 -> Out1/1
  icing/1 -> 2-D Lookup Table/2, 2-D Lookup Table6/2, 2-D Lookup Table7/2, 2-D Lookup Table8/2, 2-D Lookup Table4/2, 2-D Lookup Table5/2, 2-D Lookup Table3/2, 2-D Lookup Table2/2, 2-D Lookup Table1/2
  2-D Lookup Table1/1 -> Mux/2
  beta/1 -> 2-D Lookup Table5/1, 2-D Lookup Table8/1, 2-D Lookup Table7/1, 2-D Lookup Table6/1, 2-D Lookup Table4/1, 2-D Lookup Table3/1, 2-D Lookup Table2/1, 2-D Lookup Table1/1, 2-D Lookup Table/1
  2-D Lookup Table2/1 -> Mux/3
  2-D Lookup Table/1 -> Mux/1
  2-D Lookup Table5/1 -> Mux/5
  2-D Lookup Table3/1 -> Mux/4
  2-D Lookup Table4/1 -> Mux/6
  2-D Lookup Table6/1 -> Mux/7
  2-D Lookup Table7/1 -> Mux/8
  2-D Lookup Table8/1 -> Mux/9

== matlab function X8_trim/Subsystem/Forces/MATLAB Function ==
  settings: updateMethod=CONTINUOUS
  data: states input; tau output; wind input; control input; P parameter; Va output; alpha output; beta output; course output; crab output; gamma output; gamma_a output; wind_x output; wind_y output; wind_z output; prop_torque output; stabilityParams input; controlParams input
function [tau,Va, alpha, beta, course, crab, gamma, gamma_a, wind_x,wind_y,wind_z,prop_torque]  = fcn(states,wind,control,P, stabilityParams,controlParams)
%#codegen
% ,Va, alpha, beta, course, crab, gamma, gamma_a, wind_b,T_prop
quat = [states.Quaternion.ScalarPart,states.Quaternion.VectorPart']';
if abs(quatnorm(quat')-1)>1e-6
    quat = quatnormalize(quat');
    states.Quaternion.ScalarPart = quat(1);
    states.Quaternion.VectorPart(1) = quat(2);
    states.Quaternion.VectorPart(2) = quat(3);
    states.Quaternion.VectorPart(3) = quat(4);
end
temp = forces([states.Position.p_N,states.Position.p_E,states.Position.p_D,                     ...
               states.Attitude.phi,states.Attitude.theta,states.Attitude.psi]',                 ...
              [states.Velocity.u,states.Velocity.v,states.Velocity.w,                           ...
               states.AngularVelocity.p,states.AngularVelocity.q,states.AngularVelocity.r]',    ...
              [states.Quaternion.ScalarPart;states.Quaternion.VectorPart]',                     ...
               control,                                                                         ...
               wind,                                                                            ...
               P,                                                                               ...
               0,    ...    
               stabilityParams, ... 
               controlParams, ...
           0);
       tau = temp(1:6);
% AirData.Va      = temp(7);
% AirData.alpha   = temp(8);
% AirData.beta    = temp(9);
% AirData.course  = temp(10);
% AirData.crab    = temp(11);
% AirData.gamma   = temp(12);
% AirData.gamma_a = temp(13);
% AirData.wind_x  = temp(14);
% AirData.wind_y  = temp(15);
% AirData.wind_z  = temp(16);
Va      = temp(7);
alpha   = temp(8);
beta    = temp(9);
course  = temp(10);
crab    = temp(11);
gamma   = temp(12);
gamma_a = temp(13);
wind_x  = temp(14);
wind_y  = temp(15);
wind_z  = temp(16);
prop_torque     = temp(17);

== matlab function X8_trim/Subsystem/Dynamics1/q2euler ==
  data: scalar input; phi output; theta output; psi output; vect input
function [phi,theta,psi] = fcn(scalar,vect)
%#codegen
q = [scalar,vect']';
if abs(quatnorm(q')-1)>1e-6
    q = quatnormalize(q')';
end
[phi,theta,psi] = q2euler(q');
end

== matlab function X8_trim/Subsystem/Dynamics1/dynamics ==
  settings: updateMethod=CONTINUOUS
  data: states input; tau input size=6; y output; P parameter
function y = fcn(states,tau, P)
%#codegen

% states.Position
% states.Quaternion.ScalarPart
% states.Quaternion.VectorPart(1)
% states.Quaternion.VectorPart(2)
% states.Quaternion.VectorPart(3)
% states.Velocity
% states.AngularVelocity

quat = [states.Quaternion.ScalarPart,states.Quaternion.VectorPart']';
if abs(quatnorm(quat')-1)>1e-6
    quat = quatnormalize(quat');
    states.Quaternion.ScalarPart = quat(1);
    states.Quaternion.VectorPart(1) = quat(2);
    states.Quaternion.VectorPart(2) = quat(3);
    states.Quaternion.VectorPart(3) = quat(4);
end
y = dynamics([states.Position.p_N,states.Position.p_E,states.Position.p_D]',[states.Quaternion.ScalarPart,states.Quaternion.VectorPart']',...
       [states.Velocity.u,states.Velocity.v,states.Velocity.w]',[states.AngularVelocity.p,states.AngularVelocity.q,states.AngularVelocity.r]',...
       tau,P);
% 
% if quatnorm(states(4:7)')
% y = dynamics(states(1:3),states(4:7),states(8:10),states(11:13),tau,P);
end

== matlab function X8_trim/Subsystem/Dynamics1/MATLAB Function ==
  data: q input; scalar output; vect output
function [scalar, vect] = fcn(q)
%#codegen

q_normal = q/norm(q);
% disp(norm(q_normal)-1)
scalar = q_normal(1);
vect = q_normal(2:4);
end

== matlab function X8_trim/Subsystem/Forces/MATLAB Function1 ==
  settings: updateMethod=CONTINUOUS
  data: states input; alpha output; wind input; beta output
function [alpha,beta] = fcn(states,wind)
v_b = [states.Velocity.u,states.Velocity.v,states.Velocity.w]';
v_r = v_b - wind(1:3);
alpha = atan2(v_r(3),v_r(1));
beta = asin(v_r(2)/sqrt(v_r(1)^2 + v_r(2)^2 + v_r(3)^2));

end
